simulink model "Ex3"  (R2020a)
settings: Solver=VariableStepAuto  StartTime=0.0  StopTime=.2  MaxStep=10^-5  RelTol=1e-3
InitFcn:
  | Alpha=45;
libraries: powerlib x16
settings Model: Creator=User  LastModifiedBy=User

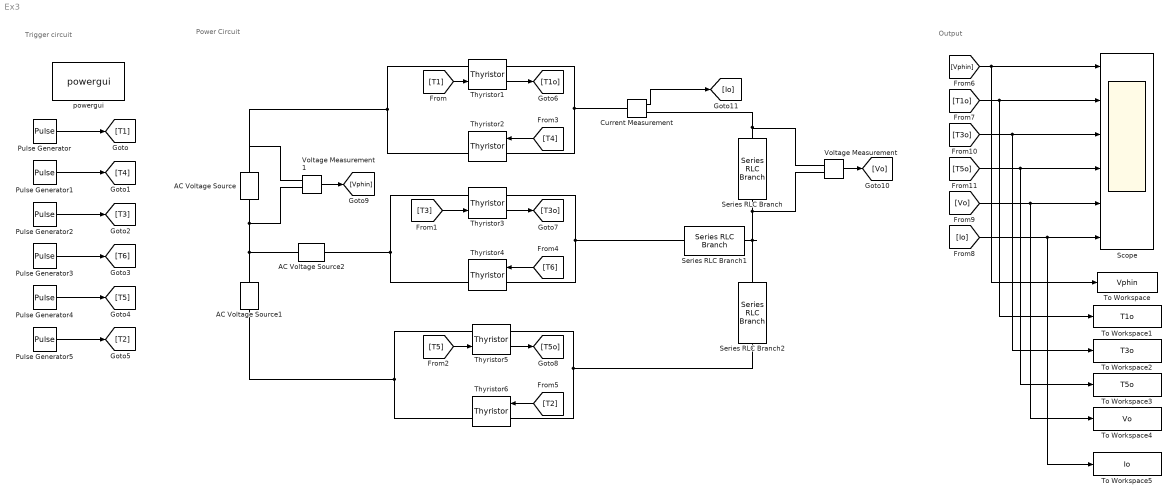
== system Ex3 ==
  note: Output
  note: Power Circuit
  note: Trigger circuit
  AC Voltage Source : powerlib/Electrical Sources/AC Voltage Source  Amplitude=380  Phase=0  Frequency=50  SampleTime=0  Measurements=None  BusType=swing  Pref=10e3  Qref=0  Qmin=-inf  Qmax=+inf
  AC Voltage Source1 : powerlib/Electrical Sources/AC Voltage Source  Amplitude=380  Phase=120  Frequency=50  SampleTime=0  Measurements=None  BusType=swing  Pref=10e3  Qref=0  Qmin=-inf  Qmax=+inf
  AC Voltage Source2 : powerlib/Electrical Sources/AC Voltage Source  Amplitude=380  Phase=240  Frequency=50  SampleTime=0  Measurements=None  BusType=swing  Pref=10e3  Qref=0  Qmin=-inf  Qmax=+inf
  Current Measurement : powerlib/Measurements/Current Measurement  PhasorSimulation=off  OutputType=Complex  PSBequivalent=0
  Pulse Generator : DiscretePulseGenerator  PulseType=Time based  Period=.02  PulseWidth=5  PhaseDelay=Alpha*(1/(50*360))
  Pulse Generator1 : DiscretePulseGenerator  PulseType=Time based  Period=.02  PulseWidth=5  PhaseDelay=(Alpha+180)*(1/(50*360))
  Pulse Generator2 : DiscretePulseGenerator  PulseType=Time based  Period=.02  PulseWidth=5  PhaseDelay=(Alpha+120)*(1/(50*360))
  Pulse Generator3 : DiscretePulseGenerator  PulseType=Time based  Period=.02  PulseWidth=5  PhaseDelay=(Alpha+180+120)*(1/(50*360))
  Pulse Generator4 : DiscretePulseGenerator  PulseType=Time based  Period=.02  PulseWidth=5  PhaseDelay=(Alpha+240)*(1/(50*360))
  Pulse Generator5 : DiscretePulseGenerator  PulseType=Time based  Period=.02  PulseWidth=5  PhaseDelay=(Alpha+180+240)*(1/(50*360))
  Scope : Scope  NumInputPorts=6
  Series RLC Branch : powerlib/Elements/Series RLC Branch  LConnTagsString=__new0  RConnTagsString=__new0  BranchType=R  Resistance=10  Inductance=1e-3  SetiL0=off  InitialCurrent=0  Capacitance=1e-6  Setx0=off  InitialVoltage=0  Measurements=None
  Series RLC Branch1 : powerlib/Elements/Series RLC Branch  LConnTagsString=__new0  RConnTagsString=__new0  BranchType=R  Resistance=10  Inductance=1e-3  SetiL0=off  InitialCurrent=0  Capacitance=1e-6  Setx0=off  InitialVoltage=0  Measurements=None
  Series RLC Branch2 : powerlib/Elements/Series RLC Branch  LConnTagsString=__new0  RConnTagsString=__new0  BranchType=R  Resistance=10  Inductance=1e-3  SetiL0=off  InitialCurrent=0  Capacitance=1e-6  Setx0=off  InitialVoltage=0  Measurements=None
  Thyristor{1..6} (6 alike) : powerlib/Power Electronics/Thyristor  Ron=0.001  Lon=0  Vf=0.8  IC=0  Rs=500  Cs=250e-9  Measurements=on
  To Workspace : ToWorkspace  VariableName=Vphin  SampleTime=-1
  To Workspace1 : ToWorkspace  VariableName=T1o  SaveFormat=Timeseries  SampleTime=-1
  To Workspace2 : ToWorkspace  VariableName=T3o  SaveFormat=Timeseries  SampleTime=-1
  To Workspace3 : ToWorkspace  VariableName=T5o  SaveFormat=Timeseries  SampleTime=-1
  To Workspace4 : ToWorkspace  VariableName=Vo  SampleTime=-1
  To Workspace5 : ToWorkspace  VariableName=Io  SampleTime=-1
  Voltage Measurement : powerlib/Measurements/Voltage Measurement  PhasorSimulation=off  OutputType=Complex  PSBequivalent=0
  Voltage Measurement1 : powerlib/Measurements/Voltage Measurement  PhasorSimulation=off  OutputType=Complex  PSBequivalent=0
  powergui : powerlib/powergui  Priority=1  SimulationMode=Continuous  SampleTime=50e-6  frequency=60  Iterations=50  frequencyindice=50  Pbase=100e6  ErrMax=1e-4  UnitsV=kV  UnitsW=MW  buscounter=0  FunctionMessages=off  echomessages=off  EnableUseOfTLC=off  CurrentSourceSwitches=off  DisableSnubberDevices=on  DisableRonSwitches=on  DisableVfSwitches=on  DisplayEquations=off  AutomaticDiscreteSolvers=off  SolverType=Tustin/Backward Euler (TBE)  Interpol=off  ExternalGateDelay=off  methode=off  Ts=100  x0status=blocks  SPID=on  SwTol=0  HookPort=off  NonlinearTolerance=1e-4  nMaxIteration=100  ContinueOnMaxIteration=off  RestoreLinks=warning  ResistiveCurrentMeasurement=off  Frange=[0:2:500]  Ylog=off  Xlog=on  ShowGrid=off  save=off  variable=ZData  structure=0  ZoomFFT=off  StartTime=0.0  cycles=1  DisplayStyle=1  fundamental=60  FreqAxis=off  MaxFrequency=1000  frequencyindicesteady=1  RmsSteady=1  display=off
  wires:
  Pulse Generator/1 -> [T1]
  Pulse Generator1/1 -> [T4]
  Pulse Generator5/1 -> [T2]
  Pulse Generator4/1 -> [T5]
  Pulse Generator3/1 -> [T6]
  Pulse Generator2/1 -> [T3]
  [T1] -> Thyristor1/1
  [T3] -> Thyristor3/1
  [T5] -> Thyristor5/1
  [T4] -> Thyristor2/1
  [T6] -> Thyristor4/1
  [T2] -> Thyristor6/1
  Thyristor1/1 -> [T1o]
  Thyristor3/1 -> [T3o]
  Thyristor5/1 -> [T5o]
  Voltage Measurement1/1 -> [Vphin]
  Voltage Measurement/1 -> [Vo]
  Current Measurement/1 -> [Io]
  [Vphin] -> To Workspace/1, Scope/1
  [T1o] -> To Workspace1/1, Scope/2
  [T3o] -> To Workspace2/1, Scope/3
  [T5o] -> To Workspace3/1, Scope/4
  [Vo] -> To Workspace4/1, Scope/5
  [Io] -> To Workspace5/1, Scope/6
  connections:
  AC Voltage Source1/LConn1 -- AC Voltage Source/LConn1 -- Voltage Measurement1/LConn2 -- AC Voltage Source2/LConn1
  Thyristor1/LConn1 -- Voltage Measurement1/LConn1 -- AC Voltage Source/RConn1 -- Thyristor2/RConn1
  Thyristor1/RConn1 -- Current Measurement/LConn1 -- Thyristor2/LConn1
  Thyristor3/LConn1 -- AC Voltage Source2/RConn1 -- Thyristor4/RConn1
  Thyristor3/RConn1 -- Thyristor4/LConn1 -- Series RLC Branch1/LConn1
  Thyristor5/LConn1 -- Thyristor6/RConn1 -- AC Voltage Source1/RConn1
  Thyristor5/RConn1 -- Thyristor6/LConn1 -- Series RLC Branch2/RConn1
  Series RLC Branch/LConn1 -- Current Measurement/RConn1 -- Voltage Measurement/LConn1
  Series RLC Branch1/RConn1 -- Series RLC Branch2/LConn1 -- Voltage Measurement/LConn2 -- Series RLC Branch/RConn1
